simulink model "Factorial_WhileLoop"  (R2021a)
settings: Solver=FixedStepDiscrete  StartTime=0.0  StopTime=10.0  RelTol=1e-3
settings Model: Creator=Moamen_Hamed  LastModifiedBy=AL_hamd
settings OptimizationCC: DefaultParameterBehavior=Inlined  EnhancedBackFolding=on  PassReuseOutputArgsAs=Individual arguments  OptimizeBlockOrder=speed  DifferentSizesBufferReuse=on  OptimizationCustomize=off  EfficientTunableParamExpr=on
settings DebuggingCC: ParameterTunabilityLossMsg=error
settings SFSimCC: MATLABDynamicMemAlloc=off
settings RTWCC: SystemTargetFile=ert.tlc  GenCodeOnly=on  TemplateMakefile=ert_default_tmf  GenerateReport=on  IncludeHyperlinkInReport=on  LaunchReport=on  GenerateTraceInfo=on
settings CodeAppCC: ForceParamTrailComments=on  IgnoreCustomStorageClasses=off  OperatorAnnotations=on  SimulinkDataObjDesc=on  SFDataObjDesc=on  InsertBlockDesc=on
settings ERTTargetCC: TargetLangStandard=C99 (ISO)  GenerateSampleERTMain=on  CodeInterfacePackaging=Reusable function  SupportComplex=off  InlinedParameterPlacement=NonHierarchical  ERTCustomFileTemplate=example_file_process.tlc

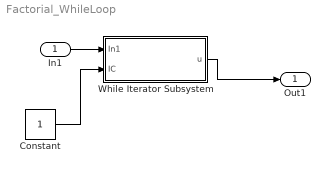
== system Factorial_WhileLoop ==
  In1 : Inport
  Constant : Constant  OutDataTypeStr=int32
  While Iterator Subsystem : Subsystem  TreatAsAtomicUnit=on
  Out1 : Outport
  wires:
  Constant/1 -> While Iterator Subsystem/2(IC)
  In1/1 -> While Iterator Subsystem/1(In1)
  While Iterator Subsystem/1(u) -> Out1/1

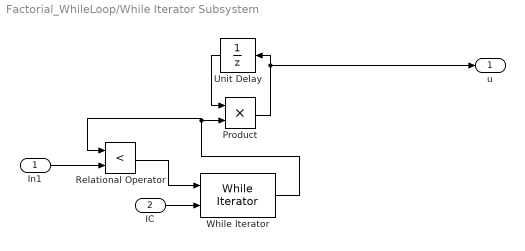
== system Factorial_WhileLoop/While Iterator Subsystem ==
  In1 : Inport
  IC : Inport  Port=2
  Product : Product  OutDataTypeStr=int32
  Relational Operator : RelationalOperator  Operator=<  OutDataTypeStr=boolean  RndMeth=Simplest
  Unit Delay : UnitDelay  InitialCondition=1  SampleTime=-1  HasFrameUpgradeWarning=on
  While Iterator : WhileIterator  MaxIters=20  ShowIterationPort=on
  u : Outport
  wires:
  IC/1 -> While Iterator/2
  Relational Operator/1 -> While Iterator/1
  In1/1 -> Relational Operator/2
  Product/1 -> u/1, Unit Delay/1
  Unit Delay/1 -> Product/1
  While Iterator/1 -> Relational Operator/1, Product/2
